simulink library "sm_trackV_lib_chain_contact"  (R2026a)
settings: Solver=VariableStepAuto
undefined symbols (not defined in the file): Excv
libraries: sm_lib x9
Description:
  | Copyright 2024-2026 The MathWorks, Inc.
settings Model: Creator=smiller  LastModifiedBy=smiller

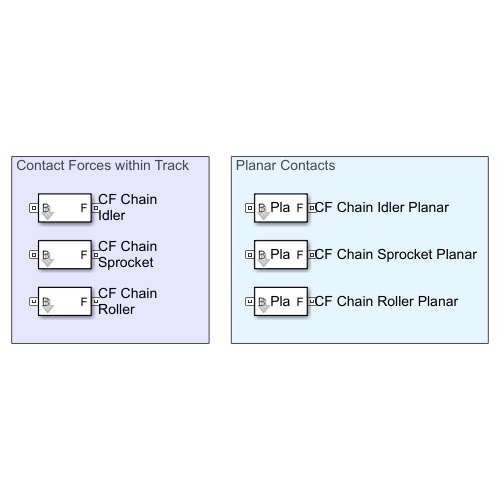
[thumbnail: Simulink's stored preview of the top-level diagram]
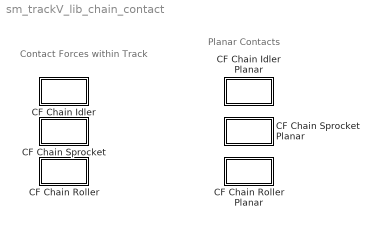
== system sm_trackV_lib_chain_contact ==
  note: Contact Forces within Track
  note: Planar Contacts
  CF Chain Idler : Subsystem  mask(Contact Force Between Chain and Idler){NormalStiffness=Excv.Contact.Idler.K, NormalDamping=Excv.Contact.Idler.B, NormalTransitionRegionWidth=Excv.Contact.Idler.TW}
      mask prompts: NormalStiffness "Normal Stiffness (N/m)"; NormalDamping "Normal Damping (N/(m/s))"; NormalTransitionRegionWidth "Normal Transition Width (m)"
      mask help: Models contact force between one link of the chain and idler.
      mask TypeOptions NormalStiffness:
      | Spatial
      | Contact Force/NormalStiffness
      mask TypeOptions NormalDamping:
      | Spatial
      | Contact Force/NormalDamping
      mask TypeOptions NormalTransitionRegionWidth:
      | Spatial
      | Contact Force/NormalTransitionRegionWidth
  CF Chain Roller : Subsystem  mask(Contact Force between Chain and Roller){NormalStiffness=Excv.Contact.Roller.K, NormalDamping=Excv.Contact.Roller.B, NormalTransitionRegionWidth=Excv.Contact.Roller.TW}
      mask prompts: NormalStiffness "Normal Stiffness (N/m)"; NormalDamping "Normal Damping (N/(m/s))"; NormalTransitionRegionWidth "Normal Transition Width (m)"
      mask help: Models contact force between one chain link and one roller.
      mask TypeOptions NormalStiffness:
      | Spatial
      | Contact Force/NormalStiffness
      mask TypeOptions NormalDamping:
      | Spatial
      | Contact Force/NormalDamping
      mask TypeOptions NormalTransitionRegionWidth:
      | Spatial
      | Contact Force/NormalTransitionRegionWidth
  CF Chain Sprocket : Subsystem  mask(Contact Force Between Chain and Sprocket){NormalStiffness=Excv.Contact.Sprocket.K, NormalDamping=Excv.Contact.Sprocket.B, NormalTransitionRegionWidth=Excv.Contact.Sprocket.TW}
      mask prompts: NormalStiffness "Normal Stiffness (N/m)"; NormalDamping "Normal Damping (N/(m/s))"; NormalTransitionRegionWidth "Normal Transition Width (m)"
      mask help: Models contact force between one chain link and the entire sprocket.
      mask TypeOptions NormalStiffness:
      | Spatial
      | Contact Force/NormalStiffness
      mask TypeOptions NormalDamping:
      | Spatial
      | Contact Force/NormalDamping
      mask TypeOptions NormalTransitionRegionWidth:
      | Spatial
      | Contact Force/NormalTransitionRegionWidth
  CF Chain Idler Planar : Subsystem  mask(Contact Force Between Chain and Idler){NormalStiffness=Excv.Contact.Idler.K, NormalDamping=Excv.Contact.Idler.B, NormalTransitionRegionWidth=Excv.Contact.Idler.TW}
      mask prompts: NormalStiffness "Normal Stiffness (N/m)"; NormalDamping "Normal Damping (N/(m/s))"; NormalTransitionRegionWidth "Normal Transition Width (m)"
      mask help: Models contact force between one link of the chain and idler.
      mask TypeOptions NormalStiffness:
      | Spatial
      | Contact Force/NormalStiffness
      mask TypeOptions NormalDamping:
      | Spatial
      | Contact Force/NormalDamping
      mask TypeOptions NormalTransitionRegionWidth:
      | Spatial
      | Contact Force/NormalTransitionRegionWidth
      mask Display: disp('Pla');
  CF Chain Roller Planar : Subsystem  mask(Contact Force between Chain and Roller){NormalStiffness=Excv.Contact.Roller.K, NormalDamping=Excv.Contact.Roller.B, NormalTransitionRegionWidth=Excv.Contact.Roller.TW}
      mask prompts: NormalStiffness "Normal Stiffness (N/m)"; NormalDamping "Normal Damping (N/(m/s))"; NormalTransitionRegionWidth "Normal Transition Width (m)"
      mask help: Models contact force between one chain link and one roller.
      mask TypeOptions NormalStiffness:
      | Spatial
      | Contact Force/NormalStiffness
      mask TypeOptions NormalDamping:
      | Spatial
      | Contact Force/NormalDamping
      mask TypeOptions NormalTransitionRegionWidth:
      | Spatial
      | Contact Force/NormalTransitionRegionWidth
      mask Display: disp('Pla');
  CF Chain Sprocket Planar : Subsystem  mask(Contact Force Between Chain and Sprocket){NormalStiffness=Excv.Contact.Sprocket.K, NormalDamping=Excv.Contact.Sprocket.B, NormalTransitionRegionWidth=Excv.Contact.Sprocket.TW}
      mask prompts: NormalStiffness "Normal Stiffness (N/m)"; NormalDamping "Normal Damping (N/(m/s))"; NormalTransitionRegionWidth "Normal Transition Width (m)"
      mask help: Models contact force between one chain link and the entire sprocket.
      mask TypeOptions NormalStiffness:
      | Spatial
      | Contact Force/NormalStiffness
      mask TypeOptions NormalDamping:
      | Spatial
      | Contact Force/NormalDamping
      mask TypeOptions NormalTransitionRegionWidth:
      | Spatial
      | Contact Force/NormalTransitionRegionWidth
      mask Display: disp('Pla');

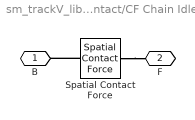
== system sm_trackV_lib_chain_contact/CF Chain Idler ==
  Spatial Contact Force : sm_lib/Forces and Torques/Spatial Contact Force  SenseSeparationDistance=off  NormalForceType=SmoothSpringDamper  NormalStiffness=NormalStiffness  NormalStiffnessUnits=N/m  NormalDamping=NormalDamping  NormalDampingUnits=N/(m/s)  NormalTransitionRegionWidth=NormalTransitionRegionWidth  NormalTransitionRegionWidthUnits=m  FrictionType=None  CoefficientOfStaticFriction=0.5  CoefficientOfDynamicFriction=0.5  FrictionalCriticalVelocity=1e-4  FrictionalCriticalVelocityUnits=m/s  SenseContactSignal=off  SensePenetrationDepth=off  SenseNormalVelocity=off  SenseTangentialVelocity=off  SensingForceTorqueDirection=BaseOnFollower  SensingForceTorqueResolutionFrame=ContactFrame  SenseNormalForce=off  SenseNormalForceMagnitude=off  SenseNormalTorque=off  SenseFrictionalForce=off  SenseFrictionalForceMagnitude=off  SenseFrictionalTorque=off  SenseTotalForce=off  SenseTotalTorque=off  SenseContactBaseRotation=off  SenseContactBaseTranslation=off  SenseContactFollowerRotation=off  SenseContactFollowerTranslation=off  ZeroCrossDetectContactStartAndEnd=off
  B : PMIOPort  Side=Left
  F : PMIOPort  Port=2  Side=Right
  connections:
  Spatial Contact Force/LConn1 -- B/RConn1
  Spatial Contact Force/RConn1 -- F/RConn1

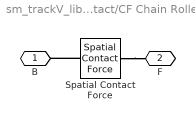
== system sm_trackV_lib_chain_contact/CF Chain Roller ==
  Spatial Contact Force : sm_lib/Forces and Torques/Spatial Contact Force  SenseSeparationDistance=off  NormalForceType=SmoothSpringDamper  NormalStiffness=NormalStiffness  NormalStiffnessUnits=N/m  NormalDamping=NormalDamping  NormalDampingUnits=N/(m/s)  NormalTransitionRegionWidth=NormalTransitionRegionWidth  NormalTransitionRegionWidthUnits=m  FrictionType=None  CoefficientOfStaticFriction=0.5  CoefficientOfDynamicFriction=0.5  FrictionalCriticalVelocity=1e-4  FrictionalCriticalVelocityUnits=m/s  SenseContactSignal=off  SensePenetrationDepth=off  SenseNormalVelocity=off  SenseTangentialVelocity=off  SensingForceTorqueDirection=BaseOnFollower  SensingForceTorqueResolutionFrame=ContactFrame  SenseNormalForce=off  SenseNormalForceMagnitude=off  SenseNormalTorque=off  SenseFrictionalForce=off  SenseFrictionalForceMagnitude=off  SenseFrictionalTorque=off  SenseTotalForce=off  SenseTotalTorque=off  SenseContactBaseRotation=off  SenseContactBaseTranslation=off  SenseContactFollowerRotation=off  SenseContactFollowerTranslation=off  ZeroCrossDetectContactStartAndEnd=off
  B : PMIOPort  Side=Left
  F : PMIOPort  Port=2  Side=Right
  connections:
  Spatial Contact Force/LConn1 -- B/RConn1
  Spatial Contact Force/RConn1 -- F/RConn1

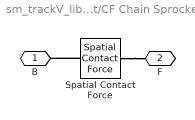
== system sm_trackV_lib_chain_contact/CF Chain Sprocket ==
  Spatial Contact Force : sm_lib/Forces and Torques/Spatial Contact Force  SenseSeparationDistance=off  NormalForceType=SmoothSpringDamper  NormalStiffness=NormalStiffness  NormalStiffnessUnits=N/m  NormalDamping=NormalDamping  NormalDampingUnits=N/(m/s)  NormalTransitionRegionWidth=NormalTransitionRegionWidth  NormalTransitionRegionWidthUnits=m  FrictionType=None  CoefficientOfStaticFriction=0.5  CoefficientOfDynamicFriction=0.5  FrictionalCriticalVelocity=1e-4  FrictionalCriticalVelocityUnits=m/s  SenseContactSignal=off  SensePenetrationDepth=off  SenseNormalVelocity=off  SenseTangentialVelocity=off  SensingForceTorqueDirection=BaseOnFollower  SensingForceTorqueResolutionFrame=ContactFrame  SenseNormalForce=off  SenseNormalForceMagnitude=off  SenseNormalTorque=off  SenseFrictionalForce=off  SenseFrictionalForceMagnitude=off  SenseFrictionalTorque=off  SenseTotalForce=off  SenseTotalTorque=off  SenseContactBaseRotation=off  SenseContactBaseTranslation=off  SenseContactFollowerRotation=off  SenseContactFollowerTranslation=off  ZeroCrossDetectContactStartAndEnd=off
  B : PMIOPort  Side=Left
  F : PMIOPort  Port=2  Side=Right
  connections:
  Spatial Contact Force/RConn1 -- F/RConn1
  Spatial Contact Force/LConn1 -- B/RConn1

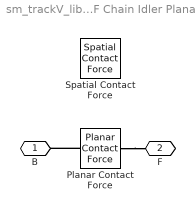
== system sm_trackV_lib_chain_contact/CF Chain Idler Planar ==
  Planar Contact Force : sm_lib/Forces and Torques/Planar Contact Force  NormalForceType=SmoothSpringDamper  NormalStiffness=NormalStiffness  NormalStiffnessUnits=N/m  NormalDamping=NormalDamping  NormalDampingUnits=N/(m/s)  NormalTransitionRegionWidth=NormalTransitionRegionWidth  NormalTransitionRegionWidthUnits=m  FrictionType=None  CoefficientOfStaticFriction=0.5  CoefficientOfDynamicFriction=0.3  FrictionalCriticalVelocity=1e-3  FrictionalCriticalVelocityUnits=m/s  SenseContactSignal=off  SensePenetrationDepth=off  SenseNormalVelocity=off  SenseTangentialVelocity=off  SensingForceTorqueDirection=BaseOnFollower  SensingForceTorqueResolutionFrame=ContactFrame  SenseNormalForce=off  SenseNormalForceMagnitude=off  SenseNormalTorque=off  SenseFrictionalForce=off  SenseFrictionalForceMagnitude=off  SenseFrictionalTorque=off  SenseTotalForce=off  SenseTotalTorque=off  SenseContactBaseRotation=off  SenseContactBaseTranslation=off  SenseContactFollowerRotation=off  SenseContactFollowerTranslation=off  ZeroCrossDetectContactStartAndEnd=off
  Spatial Contact Force : sm_lib/Forces and Torques/Spatial Contact Force  SenseSeparationDistance=off  NormalForceType=SmoothSpringDamper  NormalStiffness=NormalStiffness  NormalStiffnessUnits=N/m  NormalDamping=NormalDamping  NormalDampingUnits=N/(m/s)  NormalTransitionRegionWidth=NormalTransitionRegionWidth  NormalTransitionRegionWidthUnits=m  FrictionType=None  CoefficientOfStaticFriction=0.5  CoefficientOfDynamicFriction=0.5  FrictionalCriticalVelocity=1e-4  FrictionalCriticalVelocityUnits=m/s  SenseContactSignal=off  SensePenetrationDepth=off  SenseNormalVelocity=off  SenseTangentialVelocity=off  SensingForceTorqueDirection=BaseOnFollower  SensingForceTorqueResolutionFrame=ContactFrame  SenseNormalForce=off  SenseNormalForceMagnitude=off  SenseNormalTorque=off  SenseFrictionalForce=off  SenseFrictionalForceMagnitude=off  SenseFrictionalTorque=off  SenseTotalForce=off  SenseTotalTorque=off  SenseContactBaseRotation=off  SenseContactBaseTranslation=off  SenseContactFollowerRotation=off  SenseContactFollowerTranslation=off  ZeroCrossDetectContactStartAndEnd=off
  B : PMIOPort  Side=Left
  F : PMIOPort  Port=2  Side=Right
  connections:
  Planar Contact Force/LConn1 -- B/RConn1
  Planar Contact Force/RConn1 -- F/RConn1

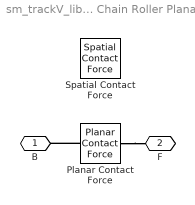
== system sm_trackV_lib_chain_contact/CF Chain Roller Planar ==
  Planar Contact Force : sm_lib/Forces and Torques/Planar Contact Force  NormalForceType=SmoothSpringDamper  NormalStiffness=NormalStiffness  NormalStiffnessUnits=N/m  NormalDamping=NormalDamping  NormalDampingUnits=N/(m/s)  NormalTransitionRegionWidth=NormalTransitionRegionWidth  NormalTransitionRegionWidthUnits=m  FrictionType=None  CoefficientOfStaticFriction=0.5  CoefficientOfDynamicFriction=0.3  FrictionalCriticalVelocity=1e-3  FrictionalCriticalVelocityUnits=m/s  SenseContactSignal=off  SensePenetrationDepth=off  SenseNormalVelocity=off  SenseTangentialVelocity=off  SensingForceTorqueDirection=BaseOnFollower  SensingForceTorqueResolutionFrame=ContactFrame  SenseNormalForce=off  SenseNormalForceMagnitude=off  SenseNormalTorque=off  SenseFrictionalForce=off  SenseFrictionalForceMagnitude=off  SenseFrictionalTorque=off  SenseTotalForce=off  SenseTotalTorque=off  SenseContactBaseRotation=off  SenseContactBaseTranslation=off  SenseContactFollowerRotation=off  SenseContactFollowerTranslation=off  ZeroCrossDetectContactStartAndEnd=off
  Spatial Contact Force : sm_lib/Forces and Torques/Spatial Contact Force  SenseSeparationDistance=off  NormalForceType=SmoothSpringDamper  NormalStiffness=NormalStiffness  NormalStiffnessUnits=N/m  NormalDamping=NormalDamping  NormalDampingUnits=N/(m/s)  NormalTransitionRegionWidth=NormalTransitionRegionWidth  NormalTransitionRegionWidthUnits=m  FrictionType=None  CoefficientOfStaticFriction=0.5  CoefficientOfDynamicFriction=0.5  FrictionalCriticalVelocity=1e-4  FrictionalCriticalVelocityUnits=m/s  SenseContactSignal=off  SensePenetrationDepth=off  SenseNormalVelocity=off  SenseTangentialVelocity=off  SensingForceTorqueDirection=BaseOnFollower  SensingForceTorqueResolutionFrame=ContactFrame  SenseNormalForce=off  SenseNormalForceMagnitude=off  SenseNormalTorque=off  SenseFrictionalForce=off  SenseFrictionalForceMagnitude=off  SenseFrictionalTorque=off  SenseTotalForce=off  SenseTotalTorque=off  SenseContactBaseRotation=off  SenseContactBaseTranslation=off  SenseContactFollowerRotation=off  SenseContactFollowerTranslation=off  ZeroCrossDetectContactStartAndEnd=off
  B : PMIOPort  Side=Left
  F : PMIOPort  Port=2  Side=Right
  connections:
  Planar Contact Force/LConn1 -- B/RConn1
  Planar Contact Force/RConn1 -- F/RConn1

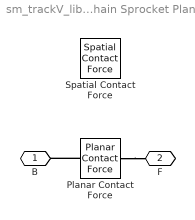
== system sm_trackV_lib_chain_contact/CF Chain Sprocket Planar ==
  Planar Contact Force : sm_lib/Forces and Torques/Planar Contact Force  NormalForceType=SmoothSpringDamper  NormalStiffness=NormalStiffness  NormalStiffnessUnits=N/m  NormalDamping=NormalDamping  NormalDampingUnits=N/(m/s)  NormalTransitionRegionWidth=NormalTransitionRegionWidth  NormalTransitionRegionWidthUnits=m  FrictionType=None  CoefficientOfStaticFriction=0.5  CoefficientOfDynamicFriction=0.3  FrictionalCriticalVelocity=1e-3  FrictionalCriticalVelocityUnits=m/s  SenseContactSignal=off  SensePenetrationDepth=off  SenseNormalVelocity=off  SenseTangentialVelocity=off  SensingForceTorqueDirection=BaseOnFollower  SensingForceTorqueResolutionFrame=ContactFrame  SenseNormalForce=off  SenseNormalForceMagnitude=off  SenseNormalTorque=off  SenseFrictionalForce=off  SenseFrictionalForceMagnitude=off  SenseFrictionalTorque=off  SenseTotalForce=off  SenseTotalTorque=off  SenseContactBaseRotation=off  SenseContactBaseTranslation=off  SenseContactFollowerRotation=off  SenseContactFollowerTranslation=off  ZeroCrossDetectContactStartAndEnd=off
  Spatial Contact Force : sm_lib/Forces and Torques/Spatial Contact Force  SenseSeparationDistance=off  NormalForceType=SmoothSpringDamper  NormalStiffness=NormalStiffness  NormalStiffnessUnits=N/m  NormalDamping=NormalDamping  NormalDampingUnits=N/(m/s)  NormalTransitionRegionWidth=NormalTransitionRegionWidth  NormalTransitionRegionWidthUnits=m  FrictionType=None  CoefficientOfStaticFriction=0.5  CoefficientOfDynamicFriction=0.5  FrictionalCriticalVelocity=1e-4  FrictionalCriticalVelocityUnits=m/s  SenseContactSignal=off  SensePenetrationDepth=off  SenseNormalVelocity=off  SenseTangentialVelocity=off  SensingForceTorqueDirection=BaseOnFollower  SensingForceTorqueResolutionFrame=ContactFrame  SenseNormalForce=off  SenseNormalForceMagnitude=off  SenseNormalTorque=off  SenseFrictionalForce=off  SenseFrictionalForceMagnitude=off  SenseFrictionalTorque=off  SenseTotalForce=off  SenseTotalTorque=off  SenseContactBaseRotation=off  SenseContactBaseTranslation=off  SenseContactFollowerRotation=off  SenseContactFollowerTranslation=off  ZeroCrossDetectContactStartAndEnd=off
  B : PMIOPort  Side=Left
  F : PMIOPort  Port=2  Side=Right
  connections:
  Planar Contact Force/RConn1 -- F/RConn1
  Planar Contact Force/LConn1 -- B/RConn1
